simulink library "JoeDeese2"  (R2018b)
settings: Solver=VariableStepAuto  StartTime=0.0  StopTime=10.0  RelTol=1e-3
settings Model: Creator=mcobb  LastModifiedBy=mcobb

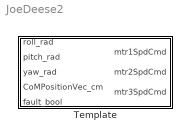
== system JoeDeese2 ==
  Template : Subsystem

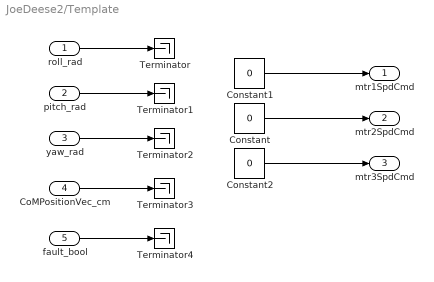
== system JoeDeese2/Template ==
  roll_rad : Inport
  pitch_rad : Inport  Port=2
  yaw_rad : Inport  Port=3
  CoMPositionVec_cm : Inport  Port=4
  fault_bool : Inport  Port=5  OutDataTypeStr=boolean
  Constant : Constant  Value=0
  Constant1 : Constant  Value=0
  Constant2 : Constant  Value=0
  Terminator{,1..4} (5 alike) : Terminator
  mtr1SpdCmd : Outport
  mtr2SpdCmd : Outport  Port=2
  mtr3SpdCmd : Outport  Port=3
  wires:
  roll_rad/1 -> Terminator/1
  pitch_rad/1 -> Terminator1/1
  yaw_rad/1 -> Terminator2/1
  CoMPositionVec_cm/1 -> Terminator3/1
  Constant/1 -> mtr2SpdCmd/1
  Constant1/1 -> mtr1SpdCmd/1
  Constant2/1 -> mtr3SpdCmd/1
  fault_bool/1 -> Terminator4/1
